simulink model "LRMate200Experimentor_Single"  (R2015b)
settings: Solver=FixedStepDiscrete  StartTime=0.0  StopTime=inf  FixedStep=si.SolverTimeStep  RelTol=1e-3  AbsTol=1e-5
undefined symbols (not defined in the file or in its folder): si
libraries: xpcethercatlib x58, slrtlib x8, xpcnilib x6
settings Model: xpc_rtwmakecfg_data=_xpcethercatlib_  SimulationMode=external  ExtModeTrigDuration=2000  ExtModeTrigDurationFloating=1000  Creator=zwashizu  LastModifiedBy=FANUC
settings SolverCC: EnableConcurrentExecution=on
settings DataIOCC: SaveFormat=Array  Refine=2
settings OptimizationCC: BlockReduction=off  OptimizeBlockIOStorage=off  BufferReuse=off  GlobalBufferReuse=off  ExpressionFolding=off  ExpressionDepthLimit=2147483647  LocalBlockOutputs=off
settings DebuggingCC: AlgebraicLoopMsg=none  ArtificialAlgebraicLoopMsg=none  UnderspecifiedInitializationDetection=Classic  MergeDetectMultiDrivingBlocksExec=none  SolverPrmCheckMsg=warning  MultiTaskDSMMsg=none  FcnCallInpInsideContextMsg=UseLocalSettings  StateNameClashWarn=warning
settings HardwareCC: ProdBitPerPointer=32  ProdLargestAtomicFloat=None  ProdWordSize=32  ProdLongLongMode=on  ProdHWDeviceType=Generic->32-bit x86 compatible
settings RTWCC: SystemTargetFile=slrt.tlc  TemplateMakefile=slrt_default_tmf  Description=Simulink Real-Time  RTWCompilerOptimization=on
settings CodeAppCC: MaxIdLength=120
settings SimulinkRealTimeCC: GeneratePreprocessorConditionals=Disable all
settings ConfigComp: CovModelRefEnable=Off  CovSFcnEnable=off

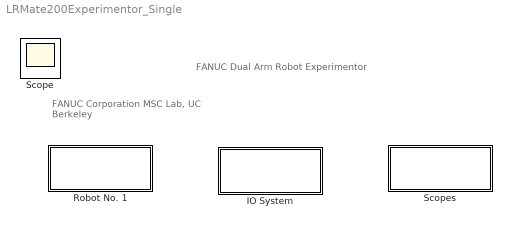
== system LRMate200Experimentor_Single ==
  note: FANUC Dual Arm Robot Experimentor
  note: FANUC Corporation
      | MSC Lab, UC Berkeley
  IO System : Subsystem
  Robot No. 1 : Subsystem
  Scopes : Subsystem
  Scope : Scope

== system LRMate200Experimentor_Single/IO System ==
  note: The Board Bus/Slot Number might be different in different TargetPC
  Button : Subsystem
  DSA System : Subsystem
  "EtherCAT Init " : xpcethercatlib/EtherCAT Init   Priority=0  config_file=F:\TeTang\V4.0\experimentor\ENI_File_20150509_2DSA.xml  device_id=0  pci_bus=3  pci_slot=0  dctuning=0  enaDebug=off  enaDC=on  errLink=off  masterDbg=off  stateChgDbg=on  baseClock=off  masterCfg=off  logFile='c:\dbglog.txt'  sample_time=0.000250
  EtherCAT Init Status : Subsystem
  Force Sensor : Subsystem
  Gripper System : Subsystem
  IO Board Brake Subsystem : Subsystem
  wires:
  "EtherCAT Init "/1 -> EtherCAT Init Status/1(In1)

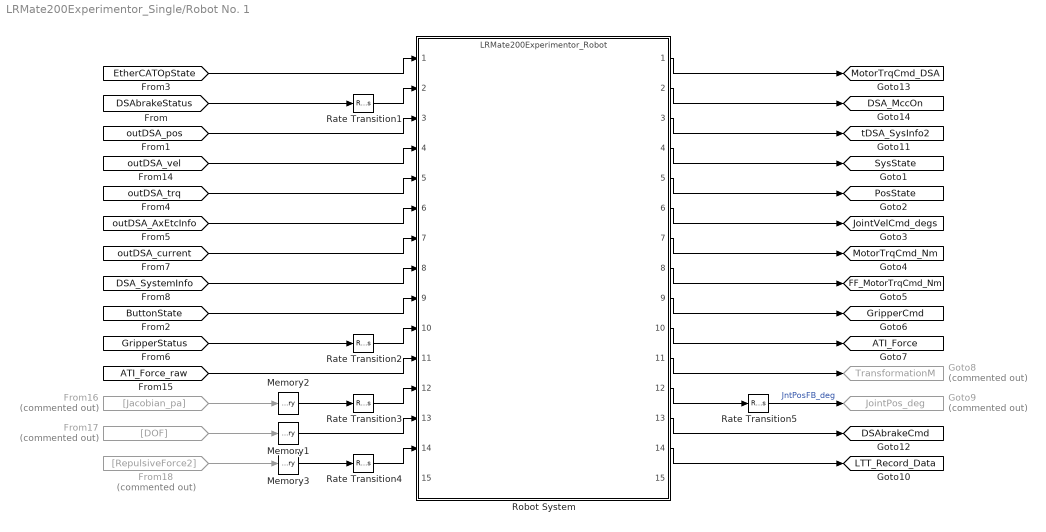
== system LRMate200Experimentor_Single/Robot No. 1 ==
  From16 : From  Commented=on  GotoTag=Jacobian_pa  TagVisibility=global
  From17 : From  Commented=on  GotoTag=DOF  TagVisibility=global
  From18 : From  Commented=on  GotoTag=RepulsiveForce2  TagVisibility=global
  Goto8 : Goto  Commented=on  GotoTag=TransformationM  TagVisibility=global
  Goto9 : Goto  Commented=on  GotoTag=JointPos_deg  TagVisibility=global
  Memory1 : Memory  InheritSampleTime=on
  Memory2 : Memory  InheritSampleTime=on
  Memory3 : Memory  InheritSampleTime=on
  Rate Transition{1..4} (4 alike) : RateTransition
  Rate Transition5 : RateTransition  OutPortSampleTime=si.tsv
  Robot System : ModelReference  ModelNameDialog=LRMate200Experimentor_Robot.slx  ParameterArgumentNames=rsi  ParameterArgumentValues=si.ri{1}  SimulationMode=Normal  ModelReferenceVersion=1.702  CopyOfModelName=LRMate200Experimentor_Robot.slx
  tag scope: ATI_Force=global, DSA_MccOn=global, DSAbrakeCmd=global, FF_MotorTrqCmd_Nm=global, GripperCmd=global, JointVelCmd_degs=global, LTT_Record_Data=global, MotorTrqCmd_DSA=global, MotorTrqCmd_Nm=global, PosState=global, SysState=global, tDSA_SysInfo2=global
  wires:
  [EtherCATOpState] -> Robot System/1
  [DSAbrakeStatus] -> Rate Transition1/1
  [outDSA_pos] -> Robot System/3
  [outDSA_vel] -> Robot System/4
  [outDSA_trq] -> Robot System/5
  [outDSA_AxEtcInfo] -> Robot System/6
  [outDSA_current] -> Robot System/7
  [DSA_SystemInfo] -> Robot System/8
  [ButtonState] -> Robot System/9
  [GripperStatus] -> Rate Transition2/1
  [ATI_Force_raw] -> Robot System/11
  From16/1 -> Memory2/1
  From17/1 -> Memory1/1
  From18/1 -> Memory3/1
  Robot System/13 -> [DSAbrakeCmd]
  Robot System/12 -> Rate Transition5/1
  Robot System/11 -> Goto8/1
  Robot System/10 -> [ATI_Force]
  Robot System/9 -> [GripperCmd]
  Robot System/8 -> [FF_MotorTrqCmd_Nm]
  Robot System/7 -> [MotorTrqCmd_Nm]
  Robot System/6 -> [JointVelCmd_degs]
  Robot System/5 -> [PosState]
  Robot System/4 -> [SysState]
  Robot System/3 -> [tDSA_SysInfo2]
  Robot System/2 -> [DSA_MccOn]
  Robot System/1 -> [MotorTrqCmd_DSA]
  Rate Transition1/1 -> Robot System/2
  Rate Transition2/1 -> Robot System/10
  Rate Transition3/1 -> Robot System/12
  Rate Transition4/1 -> Robot System/14
  Memory3/1 -> Rate Transition4/1
  Memory1/1 -> Robot System/13
  Memory2/1 -> Rate Transition3/1
  Rate Transition5/1 -> Goto9/1  "JntPosFB_deg"
  Robot System/14 -> [LTT_Record_Data]

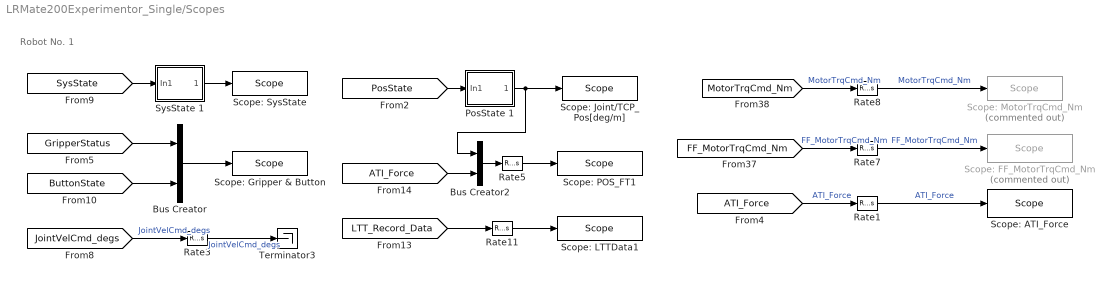
== system LRMate200Experimentor_Single/Scopes ==
  note: Robot No. 1
  Bus Creator : BusCreator  Inputs=2
  Bus Creator2 : BusCreator  Inputs=2
  PosState 1 : Subsystem
  Rate{1,3,5,7..8,11} (6 alike) : RateTransition  OutPortSampleTime=si.tsv
  Scope: ATI_Force : slrtlib/Displays and Logging/Scope   scopeno=7  scopetype=Target  autostart=on  viewmode=Graphical rolling  formatstr='%15.6f'  grid=on  ylimits=[0,0]  nosamples=40000  noprepostsamples=0  interleave=1  triggermode=FreeRun  triggersignal=1  trigsignalfromport=off  triggerlevel=0.0  triggerslope=Either  triggerscope=1  triggersample=0  filename=data.dat  mode=Lazy  writesize=512  autorestart=off  dynamicfilemode=off  maxwritefilesize=512*1024^2
  Scope: FF_MotorTrqCmd_Nm : slrtlib/Displays and Logging/Scope   Commented=on  scopeno=7  scopetype=Target  autostart=on  viewmode=Graphical rolling  formatstr='%15.6f'  grid=on  ylimits=[0,0]  nosamples=40000  noprepostsamples=0  interleave=1  triggermode=FreeRun  triggersignal=1  trigsignalfromport=off  triggerlevel=0.0  triggerslope=Either  triggerscope=1  triggersample=0  filename=data.dat  mode=Lazy  writesize=512  autorestart=off  dynamicfilemode=off  maxwritefilesize=512*1024^2
  Scope: Gripper & Button : slrtlib/Displays and Logging/Scope   scopeno=3  scopetype=Target  autostart=on  viewmode=Numerical  formatstr='%15.6f'  grid=on  ylimits=[0,0]  nosamples=10  noprepostsamples=0  interleave=1  triggermode=FreeRun  triggersignal=1  trigsignalfromport=off  triggerlevel=0.0  triggerslope=Either  triggerscope=1  triggersample=0  filename=data.dat  mode=Lazy  writesize=512  autorestart=off  dynamicfilemode=off  maxwritefilesize=512*1024^2
  Scope: Joint/TCP_Pos[deg/m] : slrtlib/Displays and Logging/Scope   scopeno=2  scopetype=Target  autostart=on  viewmode=Numerical  formatstr='%15.6f'  grid=on  ylimits=[0,0]  nosamples=100  noprepostsamples=0  interleave=1  triggermode=FreeRun  triggersignal=1  trigsignalfromport=off  triggerlevel=0.0  triggerslope=Either  triggerscope=1  triggersample=0  filename=data.dat  mode=Lazy  writesize=512  autorestart=off  dynamicfilemode=off  maxwritefilesize=512*1024^2
  Scope: LTTData1 : slrtlib/Displays and Logging/Scope   scopeno=12  scopetype=File  autostart=on  viewmode=Graphical redraw  formatstr='%15.6f'  grid=on  ylimits=[0,0]  nosamples=si.FileScope_NumberOfSamples  noprepostsamples=0  interleave=1  triggermode=FreeRun  triggersignal=1  trigsignalfromport=off  triggerlevel=0.0  triggerslope=Either  triggerscope=1  triggersample=0  filename=c:LTTData1.dat  mode=Lazy  writesize=512  autorestart=on  dynamicfilemode=off  maxwritefilesize=512*1024^2
  Scope: MotorTrqCmd_Nm : slrtlib/Displays and Logging/Scope   Commented=on  scopeno=3  scopetype=Target  autostart=on  viewmode=Graphical rolling  formatstr='%15.6f'  grid=on  ylimits=[0,0]  nosamples=40000  noprepostsamples=0  interleave=1  triggermode=FreeRun  triggersignal=1  trigsignalfromport=off  triggerlevel=0.0  triggerslope=Either  triggerscope=1  triggersample=0  filename=data.dat  mode=Lazy  writesize=512  autorestart=off  dynamicfilemode=off  maxwritefilesize=512*1024^2
  Scope: POS_FT1 : slrtlib/Displays and Logging/Scope   scopeno=10  scopetype=File  autostart=on  viewmode=Graphical redraw  formatstr='%15.6f'  grid=on  ylimits=[0,0]  nosamples=si.FileScope_NumberOfSamples  noprepostsamples=0  interleave=1  triggermode=FreeRun  triggersignal=1  trigsignalfromport=off  triggerlevel=0.0  triggerslope=Either  triggerscope=1  triggersample=0  filename=c:POS_FT1.dat  mode=Lazy  writesize=512  autorestart=on  dynamicfilemode=off  maxwritefilesize=512*1024^2
  Scope: SysState : slrtlib/Displays and Logging/Scope   scopeno=1  scopetype=Target  autostart=on  viewmode=Numerical  formatstr='%15.6f'  grid=on  ylimits=[0,0]  nosamples=10  noprepostsamples=0  interleave=1  triggermode=FreeRun  triggersignal=1  trigsignalfromport=off  triggerlevel=0.0  triggerslope=Either  triggerscope=1  triggersample=0  filename=data.dat  mode=Lazy  writesize=512  autorestart=off  dynamicfilemode=off  maxwritefilesize=512*1024^2
  SysState 1 : Subsystem
  Terminator3 : Terminator
  wires:
  [PosState] -> PosState 1/1(In1)
  [FF_MotorTrqCmd_Nm] -> Rate7/1  "FF_MotorTrqCmd_Nm"
  Rate7/1 -> Scope: FF_MotorTrqCmd_Nm/1  "FF_MotorTrqCmd_Nm"
  [MotorTrqCmd_Nm] -> Rate8/1  "MotorTrqCmd_Nm"
  Rate8/1 -> Scope: MotorTrqCmd_Nm/1  "MotorTrqCmd_Nm"
  [SysState] -> SysState 1/1(In1)
  SysState 1/1(Out1) -> Scope: SysState/1
  [ATI_Force] -> Rate1/1  "ATI_Force"
  Rate1/1 -> Scope: ATI_Force/1  "ATI_Force"
  [GripperStatus] -> Bus Creator/1
  [ButtonState] -> Bus Creator/2
  Bus Creator/1 -> Scope: Gripper & Button/1
  [JointVelCmd_degs] -> Rate3/1  "JointVelCmd_degs"
  Rate3/1 -> Terminator3/1  "JointVelCmd_degs"
  PosState 1/1(Out1) -> Scope: Joint/TCP_Pos[deg/m]/1, Bus Creator2/1
  [ATI_Force] -> Bus Creator2/2
  Bus Creator2/1 -> Rate5/1
  Rate5/1 -> Scope: POS_FT1/1
  [LTT_Record_Data] -> Rate11/1
  Rate11/1 -> Scope: LTTData1/1

== system LRMate200Experimentor_Single/IO System/Button ==
  Bus Creator : BusCreator  Inputs=2
  PCI-6528 DI Port 1 : xpcnilib/Digital Input/PCI-6528 DI  channel=[5,6]  port=B  filter=[0]  filtertime=0  sample=.001  slot=-1
  tag scope: ButtonState=global
  wires:
  PCI-6528 DI Port 1/1 -> Bus Creator/1  "Green_Button"
  PCI-6528 DI Port 1/2 -> Bus Creator/2  "LTT_Button"
  Bus Creator/1 -> [ButtonState]

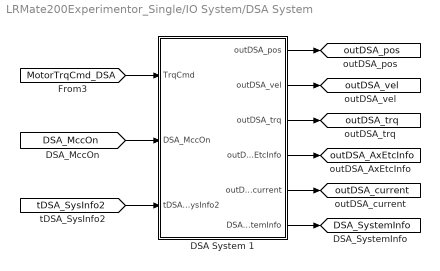
== system LRMate200Experimentor_Single/IO System/DSA System ==
  DSA System 1 : Subsystem
      settings: MinAlgLoopOccurrences=on
  tag scope: DSA_SystemInfo=global, outDSA_AxEtcInfo=global, outDSA_current=global, outDSA_pos=global, outDSA_trq=global, outDSA_vel=global
  wires:
  [MotorTrqCmd_DSA] -> DSA System 1/1(TrqCmd)
  [DSA_MccOn] -> DSA System 1/2(DSA_MccOn)
  [tDSA_SysInfo2] -> DSA System 1/3(tDSA_SysInfo2)
  DSA System 1/1(outDSA_pos) -> [outDSA_pos]
  DSA System 1/2(outDSA_vel) -> [outDSA_vel]
  DSA System 1/3(outDSA_trq) -> [outDSA_trq]
  DSA System 1/4(outDSA_AxEtcInfo) -> [outDSA_AxEtcInfo]
  DSA System 1/5(outDSA_current) -> [outDSA_current]
  DSA System 1/6(DSA_SystemInfo) -> [DSA_SystemInfo]

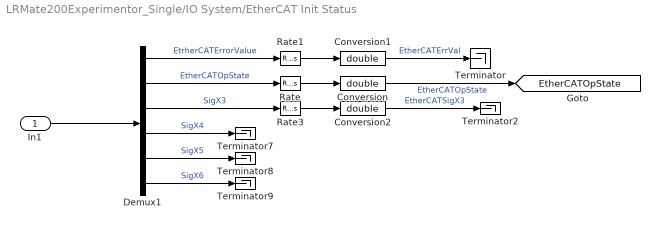
== system LRMate200Experimentor_Single/IO System/EtherCAT Init Status ==
  In1 : Inport
  Conversion : DataTypeConversion  OutDataTypeStr=double
  Conversion1 : DataTypeConversion  OutDataTypeStr=double
  Conversion2 : DataTypeConversion  OutDataTypeStr=double
  Demux1 : Demux  Outputs=6
  Rate : RateTransition  OutPortSampleTime=si.itp
  Rate1 : RateTransition  OutPortSampleTime=si.itp
  Rate3 : RateTransition  OutPortSampleTime=si.itp
  Terminator{,2,7..9} (5 alike) : Terminator
  tag scope: EtherCATOpState=global
  wires:
  Conversion2/1 -> Terminator2/1  "EtherCATSigX3"
  Demux1/4 -> Terminator7/1  "SigX4"
  Demux1/1 -> Rate1/1  "EtrherCATErrorValue"
  Demux1/3 -> Rate3/1  "SigX3"
  Demux1/5 -> Terminator8/1  "SigX5"
  Demux1/2 -> Rate/1  "EtherCATOpState"
  Rate/1 -> Conversion/1
  Rate3/1 -> Conversion2/1
  Conversion/1 -> [EtherCATOpState]  "EtherCATOpState"
  Conversion1/1 -> Terminator/1  "EtherCATErrVal"
  Rate1/1 -> Conversion1/1
  In1/1 -> Demux1/1
  Demux1/6 -> Terminator9/1  "SigX6"

== system LRMate200Experimentor_Single/IO System/Force Sensor ==
  Mux1 : Mux  Inputs=6
  PCI-6259 AD : xpcnilib/A//D/M Series/PCI-6259 AD  channel=[1,2,3,4,5,6]  range=-10*ones(1,6)  coupling=2*ones(1,6)  scantime=5e-6  sampletime=0.001  slot=-1
  tag scope: ATI_Force_raw=global
  wires:
  PCI-6259 AD/3 -> Mux1/3  "Fz(N)"
  Mux1/1 -> [ATI_Force_raw]
  PCI-6259 AD/2 -> Mux1/2  "Fy(N)"
  PCI-6259 AD/6 -> Mux1/6  "Tz(Nm)"
  PCI-6259 AD/4 -> Mux1/4  "Tx(Nm)"
  PCI-6259 AD/5 -> Mux1/5  "Ty(Nm)"
  PCI-6259 AD/1 -> Mux1/1  "Fx(N)"

== system LRMate200Experimentor_Single/IO System/Gripper System ==
  Gripper 1 : Subsystem

== system LRMate200Experimentor_Single/IO System/IO Board Brake Subsystem ==
  PCI-6528 DO : xpcnilib/Digital Output/PCI-6528 DO  channel=[1]  port=A  reset=[1]  initValue=[0]  sample=0.001  slot=-1
  Rate Transition2 : RateTransition  OutPortSampleTime=si.tsv
  tag scope: DSAbrakeStatus=global
  wires:
  [DSAbrakeCmd] -> Rate Transition2/1
  Rate Transition2/1 -> [DSAbrakeStatus], PCI-6528 DO/1  "outDSA_BrakeStatus"

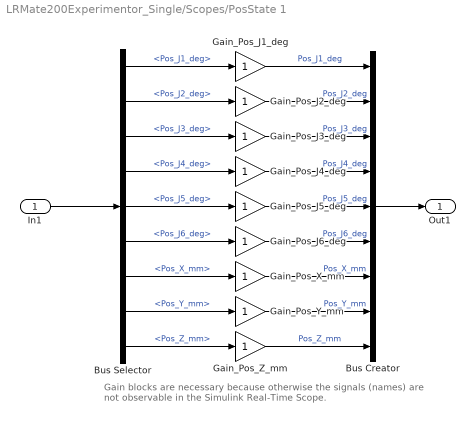
== system LRMate200Experimentor_Single/Scopes/PosState 1 ==
  note: Gain blocks are necessary because otherwise the signals (names) are not observable in the Simulink Real-Time Scope.
  In1 : Inport
  Bus Creator : BusCreator  Inputs=9
  Bus Selector : BusSelector  OutputSignals=Pos_J1_deg,Pos_J2_deg,Pos_J3_deg,Pos_J4_deg,Pos_J5_deg,Pos_J6_deg,Pos_X_mm,Pos_Y_mm,Pos_Z_mm
  Gain_Pos_J1_deg : Gain
  Gain_Pos_J2_deg : Gain
  Gain_Pos_J3_deg : Gain
  Gain_Pos_J4_deg : Gain
  Gain_Pos_J5_deg : Gain
  Gain_Pos_J6_deg : Gain
  Gain_Pos_X_mm : Gain
  Gain_Pos_Y_mm : Gain
  Gain_Pos_Z_mm : Gain
  Out1 : Outport
  wires:
  Bus Creator/1 -> Out1/1
  Bus Selector/1 -> Gain_Pos_J1_deg/1  "<Pos_J1_deg>"
  Bus Selector/2 -> Gain_Pos_J2_deg/1  "<Pos_J2_deg>"
  Bus Selector/3 -> Gain_Pos_J3_deg/1  "<Pos_J3_deg>"
  Bus Selector/4 -> Gain_Pos_J4_deg/1  "<Pos_J4_deg>"
  Bus Selector/5 -> Gain_Pos_J5_deg/1  "<Pos_J5_deg>"
  Bus Selector/6 -> Gain_Pos_J6_deg/1  "<Pos_J6_deg>"
  Bus Selector/7 -> Gain_Pos_X_mm/1  "<Pos_X_mm>"
  Bus Selector/8 -> Gain_Pos_Y_mm/1  "<Pos_Y_mm>"
  Bus Selector/9 -> Gain_Pos_Z_mm/1  "<Pos_Z_mm>"
  In1/1 -> Bus Selector/1
  Gain_Pos_J1_deg/1 -> Bus Creator/1  "Pos_J1_deg"
  Gain_Pos_J2_deg/1 -> Bus Creator/2  "Pos_J2_deg"
  Gain_Pos_J3_deg/1 -> Bus Creator/3  "Pos_J3_deg"
  Gain_Pos_J4_deg/1 -> Bus Creator/4  "Pos_J4_deg"
  Gain_Pos_J5_deg/1 -> Bus Creator/5  "Pos_J5_deg"
  Gain_Pos_J6_deg/1 -> Bus Creator/6  "Pos_J6_deg"
  Gain_Pos_X_mm/1 -> Bus Creator/7  "Pos_X_mm"
  Gain_Pos_Y_mm/1 -> Bus Creator/8  "Pos_Y_mm"
  Gain_Pos_Z_mm/1 -> Bus Creator/9  "Pos_Z_mm"

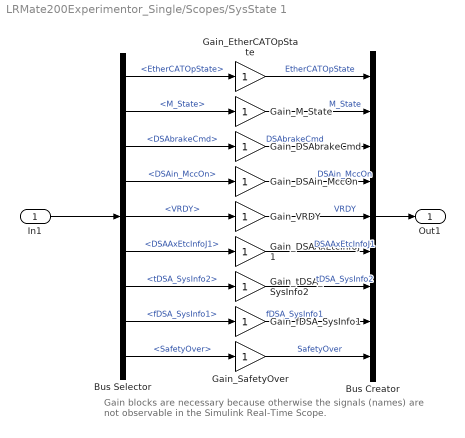
== system LRMate200Experimentor_Single/Scopes/SysState 1 ==
  note: Gain blocks are necessary because otherwise the signals (names) are not observable in the Simulink Real-Time Scope.
  In1 : Inport
  Bus Creator : BusCreator  Inputs=9
  Bus Selector : BusSelector  OutputSignals=EtherCATOpState,M_State,DSAbrakeCmd,DSAin_MccOn,VRDY,DSAAxEtcInfoJ1,tDSA_SysInfo2,fDSA_SysInfo1,SafetyOver
  Gain_DSAAxEtcInfoJ1 : Gain
  Gain_DSAbrakeCmd : Gain
  Gain_DSAin_MccOn : Gain
  Gain_EtherCATOpState : Gain
  Gain_M_State : Gain
  Gain_SafetyOver : Gain
  Gain_VRDY : Gain
  Gain_fDSA_SysInfo1 : Gain
  Gain_tDSA_SysInfo2 : Gain
  Out1 : Outport
  wires:
  Bus Creator/1 -> Out1/1
  Bus Selector/1 -> Gain_EtherCATOpState/1  "<EtherCATOpState>"
  Bus Selector/2 -> Gain_M_State/1  "<M_State>"
  Bus Selector/3 -> Gain_DSAbrakeCmd/1  "<DSAbrakeCmd>"
  Bus Selector/4 -> Gain_DSAin_MccOn/1  "<DSAin_MccOn>"
  Bus Selector/5 -> Gain_VRDY/1  "<VRDY>"
  Bus Selector/6 -> Gain_DSAAxEtcInfoJ1/1  "<DSAAxEtcInfoJ1>"
  Bus Selector/7 -> Gain_tDSA_SysInfo2/1  "<tDSA_SysInfo2>"
  Bus Selector/8 -> Gain_fDSA_SysInfo1/1  "<fDSA_SysInfo1>"
  Bus Selector/9 -> Gain_SafetyOver/1  "<SafetyOver>"
  In1/1 -> Bus Selector/1
  Gain_EtherCATOpState/1 -> Bus Creator/1  "EtherCATOpState"
  Gain_M_State/1 -> Bus Creator/2  "M_State"
  Gain_DSAbrakeCmd/1 -> Bus Creator/3  "DSAbrakeCmd"
  Gain_DSAin_MccOn/1 -> Bus Creator/4  "DSAin_MccOn"
  Gain_VRDY/1 -> Bus Creator/5  "VRDY"
  Gain_DSAAxEtcInfoJ1/1 -> Bus Creator/6  "DSAAxEtcInfoJ1"
  Gain_tDSA_SysInfo2/1 -> Bus Creator/7  "tDSA_SysInfo2"
  Gain_fDSA_SysInfo1/1 -> Bus Creator/8  "fDSA_SysInfo1"
  Gain_SafetyOver/1 -> Bus Creator/9  "SafetyOver"

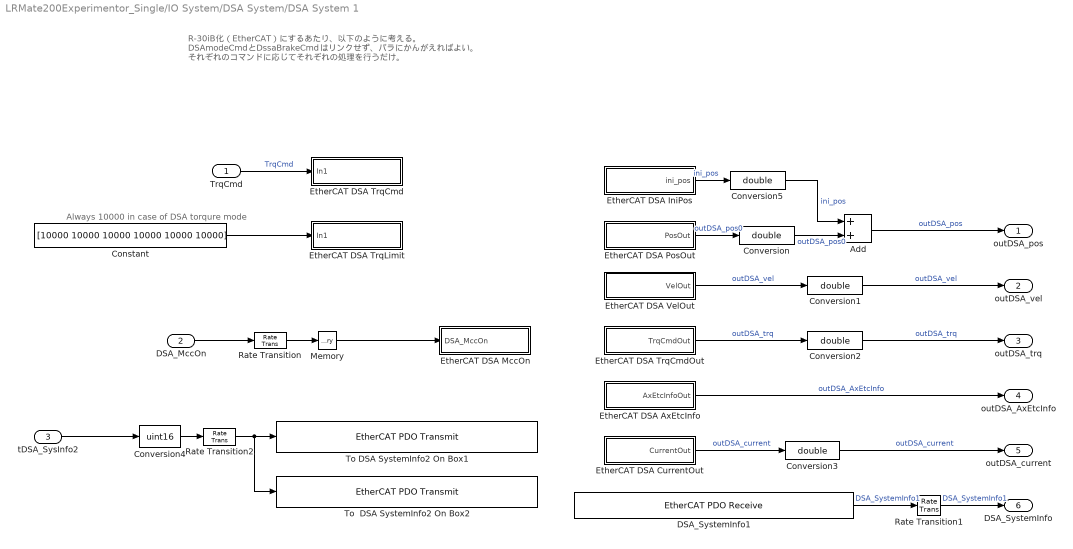
== system LRMate200Experimentor_Single/IO System/DSA System/DSA System 1 ==
  note: Always 10000 in case of DSA torqure mode
  note: R-30iB化（EtherCAT）にするあたり、以下のように考える。
      |
      | DSAmodeCmdとDssaBrakeCmdはリンクせず、パラにかんがえればよい。
      | それぞれのコマンドに応じてそれぞれの処理を行うだけ。
  TrqCmd : Inport
  DSA_MccOn : Inport  Port=2
  tDSA_SysInfo2 : Inport  Port=3
  Add : Sum
  Constant : Constant  Value=[10000 10000 10000 10000 10000 10000]  SampleTime=si.etsv
  Conversion{,1..3,5} (5 alike) : DataTypeConversion  OutDataTypeStr=double
  Conversion4 : DataTypeConversion  OutDataTypeStr=uint16
  DSA_SystemInfo1 : xpcethercatlib/EtherCAT PDO Receive  Priority=2  sig_name=Box 1 (Degital Servo Adapter).NS-IN-SYS-DCIF.NSIS01  sig_offset=1352  sig_type=uint16  type_size=16  sig_dim=1  device_id=0  sample_time=0.000250
  EtherCAT DSA AxEtcInfo : Subsystem
  EtherCAT DSA CurrentOut : Subsystem
  EtherCAT DSA IniPos : Subsystem
  EtherCAT DSA MccOn : Subsystem
  EtherCAT DSA PosOut : Subsystem
  EtherCAT DSA TrqCmd : Subsystem
  EtherCAT DSA TrqCmdOut : Subsystem
  EtherCAT DSA TrqLimit : Subsystem
  EtherCAT DSA VelOut : Subsystem
  Memory : Memory
  Rate Transition : RateTransition
  Rate Transition1 : RateTransition  OutPortSampleTime=si.tsv
  Rate Transition2 : RateTransition
  To  DSA SystemInfo2 On Box2 : xpcethercatlib/EtherCAT PDO Transmit   Priority=3  sig_name=Box 2 (Degital Servo Adapter).NS-OUT-SYS-DCIF.NSOS01  sig_offset=3656  sig_type=uint16  type_size=16  sig_dim=1  device_id=0  sample_time=0.000250
  To DSA SystemInfo2 On Box1 : xpcethercatlib/EtherCAT PDO Transmit   Priority=3  sig_name=Box 1 (Degital Servo Adapter).NS-OUT-SYS-DCIF.NSOS01  sig_offset=1352  sig_type=uint16  type_size=16  sig_dim=1  device_id=0  sample_time=0.000250
  outDSA_pos : Outport
  outDSA_vel : Outport  Port=2
  outDSA_trq : Outport  Port=3
  outDSA_AxEtcInfo : Outport  Port=4
  outDSA_current : Outport  Port=5
  DSA_SystemInfo : Outport  Port=6
  wires:
  EtherCAT DSA VelOut/1(VelOut) -> Conversion1/1  "outDSA_vel"
  EtherCAT DSA PosOut/1(PosOut) -> Conversion/1  "outDSA_pos0"
  EtherCAT DSA TrqCmdOut/1(TrqCmdOut) -> Conversion2/1  "outDSA_trq"
  EtherCAT DSA AxEtcInfo/1(AxEtcInfoOut) -> outDSA_AxEtcInfo/1  "outDSA_AxEtcInfo"
  TrqCmd/1 -> EtherCAT DSA TrqCmd/1(In1)  "TrqCmd"
  Conversion/1 -> Add/2  "outDSA_pos0"
  Conversion1/1 -> outDSA_vel/1  "outDSA_vel"
  Conversion2/1 -> outDSA_trq/1  "outDSA_trq"
  Memory/1 -> EtherCAT DSA MccOn/1(DSA_MccOn)
  Rate Transition/1 -> Memory/1
  EtherCAT DSA CurrentOut/1(CurrentOut) -> Conversion3/1  "outDSA_current"
  Conversion3/1 -> outDSA_current/1  "outDSA_current"
  DSA_MccOn/1 -> Rate Transition/1
  Rate Transition2/1 -> To  DSA SystemInfo2 On Box2/1, To DSA SystemInfo2 On Box1/1
  Conversion4/1 -> Rate Transition2/1
  tDSA_SysInfo2/1 -> Conversion4/1
  EtherCAT DSA IniPos/1(ini_pos) -> Conversion5/1  "ini_pos"
  Conversion5/1 -> Add/1  "ini_pos"
  Add/1 -> outDSA_pos/1  "outDSA_pos"
  DSA_SystemInfo1/1 -> Rate Transition1/1  "DSA_SystemInfo1"
  Constant/1 -> EtherCAT DSA TrqLimit/1(In1)
  Rate Transition1/1 -> DSA_SystemInfo/1  "DSA_SystemInfo1"

== system LRMate200Experimentor_Single/IO System/Gripper System/Gripper 1 ==
  Gripper Subsystem : Subsystem
  tag scope: GripperStatus=global
  wires:
  Gripper Subsystem/1(GripperOutput) -> [GripperStatus]
  [GripperCmd] -> Gripper Subsystem/1(GripperInput)

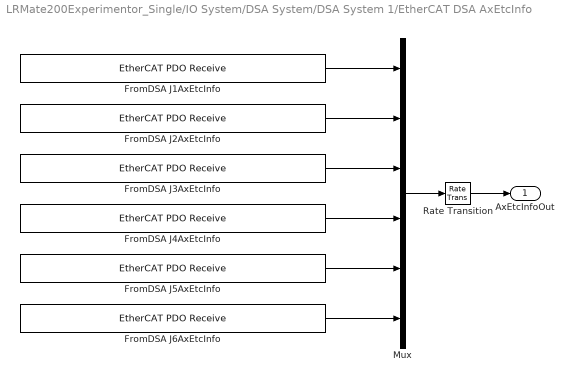
== system LRMate200Experimentor_Single/IO System/DSA System/DSA System 1/EtherCAT DSA AxEtcInfo ==
  FromDSA J1AxEtcInfo : xpcethercatlib/EtherCAT PDO Receive  Priority=2  sig_name=Box 1 (Degital Servo Adapter).NS-IN-AX01.AX01-NSI07  sig_offset=1704  sig_type=uint16  type_size=16  sig_dim=1  device_id=0  sample_time=0.000250
  FromDSA J2AxEtcInfo : xpcethercatlib/EtherCAT PDO Receive  Priority=2  sig_name=Box 1 (Degital Servo Adapter).NS-IN-AX02.AX02-NSI07  sig_offset=1896  sig_type=uint16  type_size=16  sig_dim=1  device_id=0  sample_time=0.000250
  FromDSA J3AxEtcInfo : xpcethercatlib/EtherCAT PDO Receive  Priority=2  sig_name=Box 1 (Degital Servo Adapter).NS-IN-AX03.AX03-NSI07  sig_offset=2088  sig_type=uint16  type_size=16  sig_dim=1  device_id=0  sample_time=0.000250
  FromDSA J4AxEtcInfo : xpcethercatlib/EtherCAT PDO Receive  Priority=2  sig_name=Box 1 (Degital Servo Adapter).NS-IN-AX04.AX04-NSI07  sig_offset=2280  sig_type=uint16  type_size=16  sig_dim=1  device_id=0  sample_time=0.000250
  FromDSA J5AxEtcInfo : xpcethercatlib/EtherCAT PDO Receive  Priority=2  sig_name=Box 2 (Degital Servo Adapter).NS-IN-AX01.AX01-NSI07  sig_offset=4008  sig_type=uint16  type_size=16  sig_dim=1  device_id=0  sample_time=0.000250
  FromDSA J6AxEtcInfo : xpcethercatlib/EtherCAT PDO Receive  Priority=2  sig_name=Box 2 (Degital Servo Adapter).NS-IN-AX02.AX02-NSI07  sig_offset=4200  sig_type=uint16  type_size=16  sig_dim=1  device_id=0  sample_time=0.000250
  Mux : Mux  Inputs=6
  Rate Transition : RateTransition  OutPortSampleTime=si.tsv
  AxEtcInfoOut : Outport
  wires:
  FromDSA J6AxEtcInfo/1 -> Mux/6
  FromDSA J4AxEtcInfo/1 -> Mux/4
  FromDSA J2AxEtcInfo/1 -> Mux/2
  FromDSA J5AxEtcInfo/1 -> Mux/5
  FromDSA J3AxEtcInfo/1 -> Mux/3
  FromDSA J1AxEtcInfo/1 -> Mux/1
  Mux/1 -> Rate Transition/1
  Rate Transition/1 -> AxEtcInfoOut/1

== system LRMate200Experimentor_Single/IO System/DSA System/DSA System 1/EtherCAT DSA CurrentOut ==
  FromDSA J1Current : xpcethercatlib/EtherCAT PDO Receive  Priority=2  sig_name=Box 1 (Degital Servo Adapter).HS-IN-AX01.AX01-HSI03  sig_offset=360  sig_type=int16  type_size=16  sig_dim=1  device_id=0  sample_time=0.000250
  FromDSA J2Current : xpcethercatlib/EtherCAT PDO Receive  Priority=2  sig_name=Box 1 (Degital Servo Adapter).HS-IN-AX02.AX02-HSI03  sig_offset=616  sig_type=int16  type_size=16  sig_dim=1  device_id=0  sample_time=0.000250
  FromDSA J3Current : xpcethercatlib/EtherCAT PDO Receive  Priority=2  sig_name=Box 1 (Degital Servo Adapter).HS-IN-AX03.AX03-HSI03  sig_offset=872  sig_type=int16  type_size=16  sig_dim=1  device_id=0  sample_time=0.000250
  FromDSA J4Current : xpcethercatlib/EtherCAT PDO Receive  Priority=2  sig_name=Box 1 (Degital Servo Adapter).HS-IN-AX04.AX04-HSI03  sig_offset=1128  sig_type=int16  type_size=16  sig_dim=1  device_id=0  sample_time=0.000250
  FromDSA J5Current : xpcethercatlib/EtherCAT PDO Receive  Priority=2  sig_name=Box 2 (Degital Servo Adapter).HS-IN-AX01.AX01-HSI03  sig_offset=2664  sig_type=int16  type_size=16  sig_dim=1  device_id=0  sample_time=0.000250
  FromDSA J6Current : xpcethercatlib/EtherCAT PDO Receive  Priority=2  sig_name=Box 2 (Degital Servo Adapter).HS-IN-AX02.AX02-HSI03  sig_offset=2920  sig_type=int16  type_size=16  sig_dim=1  device_id=0  sample_time=0.000250
  Mux : Mux  Inputs=6
  Rate Transition : RateTransition  OutPortSampleTime=si.tsv
  CurrentOut : Outport
  wires:
  FromDSA J6Current/1 -> Mux/6
  FromDSA J4Current/1 -> Mux/4
  FromDSA J2Current/1 -> Mux/2
  FromDSA J5Current/1 -> Mux/5
  FromDSA J3Current/1 -> Mux/3
  FromDSA J1Current/1 -> Mux/1
  Mux/1 -> Rate Transition/1
  Rate Transition/1 -> CurrentOut/1

== system LRMate200Experimentor_Single/IO System/DSA System/DSA System 1/EtherCAT DSA IniPos ==
  FromDSA J1IniPos : xpcethercatlib/EtherCAT PDO Receive  Priority=2  sig_name=Box 1 (Degital Servo Adapter).NS-IN-AX01.AX01-NSI02  sig_offset=1624  sig_type=int32  type_size=32  sig_dim=1  device_id=0  sample_time=0.000250
  FromDSA J2IniPos : xpcethercatlib/EtherCAT PDO Receive  Priority=2  sig_name=Box 1 (Degital Servo Adapter).NS-IN-AX02.AX02-NSI02  sig_offset=1816  sig_type=int32  type_size=32  sig_dim=1  device_id=0  sample_time=0.000250
  FromDSA J3IniPos : xpcethercatlib/EtherCAT PDO Receive  Priority=2  sig_name=Box 1 (Degital Servo Adapter).NS-IN-AX03.AX03-NSI02  sig_offset=2008  sig_type=int32  type_size=32  sig_dim=1  device_id=0  sample_time=0.000250
  FromDSA J4IniPos : xpcethercatlib/EtherCAT PDO Receive  Priority=2  sig_name=Box 1 (Degital Servo Adapter).NS-IN-AX04.AX04-NSI02  sig_offset=2200  sig_type=int32  type_size=32  sig_dim=1  device_id=0  sample_time=0.000250
  FromDSA J5IniPos : xpcethercatlib/EtherCAT PDO Receive  Priority=2  sig_name=Box 2 (Degital Servo Adapter).NS-IN-AX01.AX01-NSI02  sig_offset=3928  sig_type=int32  type_size=32  sig_dim=1  device_id=0  sample_time=0.000250
  FromDSA J6IniPos : xpcethercatlib/EtherCAT PDO Receive  Priority=2  sig_name=Box 2 (Degital Servo Adapter).NS-IN-AX02.AX02-NSI02  sig_offset=4120  sig_type=int32  type_size=32  sig_dim=1  device_id=0  sample_time=0.000250
  Mux : Mux  Inputs=6
  Rate Transition : RateTransition  OutPortSampleTime=si.tsv
  ini_pos : Outport
  wires:
  FromDSA J6IniPos/1 -> Mux/6
  FromDSA J4IniPos/1 -> Mux/4
  FromDSA J2IniPos/1 -> Mux/2
  FromDSA J5IniPos/1 -> Mux/5
  FromDSA J3IniPos/1 -> Mux/3
  FromDSA J1IniPos/1 -> Mux/1
  Mux/1 -> Rate Transition/1
  Rate Transition/1 -> ini_pos/1

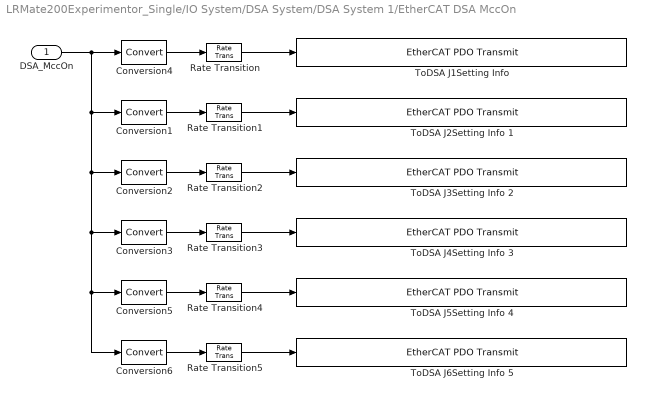
== system LRMate200Experimentor_Single/IO System/DSA System/DSA System 1/EtherCAT DSA MccOn ==
  DSA_MccOn : Inport
  Conversion{1..6} (6 alike) : DataTypeConversion
  Rate Transition{,1..5} (6 alike) : RateTransition
  "ToDSA J1Setting Info " : xpcethercatlib/EtherCAT PDO Transmit   Priority=3  sig_name=Box 1 (Degital Servo Adapter).NS-OUT-AX01.AX01-NSO03  sig_offset=1640  sig_type=uint16  type_size=16  sig_dim=1  device_id=0  sample_time=0.000250
  ToDSA J2Setting Info 1 : xpcethercatlib/EtherCAT PDO Transmit   Priority=3  sig_name=Box 1 (Degital Servo Adapter).NS-OUT-AX02.AX02-NSO03  sig_offset=1896  sig_type=uint16  type_size=16  sig_dim=1  device_id=0  sample_time=0.000250
  ToDSA J3Setting Info 2 : xpcethercatlib/EtherCAT PDO Transmit   Priority=3  sig_name=Box 1 (Degital Servo Adapter).NS-OUT-AX03.AX03-NSO03  sig_offset=2152  sig_type=uint16  type_size=16  sig_dim=1  device_id=0  sample_time=0.000250
  ToDSA J4Setting Info 3 : xpcethercatlib/EtherCAT PDO Transmit   Priority=3  sig_name=Box 1 (Degital Servo Adapter).NS-OUT-AX04.AX04-NSO03  sig_offset=2408  sig_type=uint16  type_size=16  sig_dim=1  device_id=0  sample_time=0.000250
  ToDSA J5Setting Info 4 : xpcethercatlib/EtherCAT PDO Transmit   Priority=3  sig_name=Box 2 (Degital Servo Adapter).NS-OUT-AX01.AX01-NSO03  sig_offset=3944  sig_type=uint16  type_size=16  sig_dim=1  device_id=0  sample_time=0.000250
  ToDSA J6Setting Info 5 : xpcethercatlib/EtherCAT PDO Transmit   Priority=3  sig_name=Box 2 (Degital Servo Adapter).NS-OUT-AX02.AX02-NSO03  sig_offset=4200  sig_type=uint16  type_size=16  sig_dim=1  device_id=0  sample_time=0.000250
  wires:
  Rate Transition/1 -> "ToDSA J1Setting Info "/1
  Conversion4/1 -> Rate Transition/1
  DSA_MccOn/1 -> Conversion6/1, Conversion5/1, Conversion3/1, Conversion2/1, Conversion1/1, Conversion4/1
  Rate Transition1/1 -> ToDSA J2Setting Info 1/1
  Conversion1/1 -> Rate Transition1/1
  Rate Transition2/1 -> ToDSA J3Setting Info 2/1
  Conversion2/1 -> Rate Transition2/1
  Rate Transition3/1 -> ToDSA J4Setting Info 3/1
  Conversion3/1 -> Rate Transition3/1
  Rate Transition4/1 -> ToDSA J5Setting Info 4/1
  Conversion5/1 -> Rate Transition4/1
  Rate Transition5/1 -> ToDSA J6Setting Info 5/1
  Conversion6/1 -> Rate Transition5/1

== system LRMate200Experimentor_Single/IO System/DSA System/DSA System 1/EtherCAT DSA PosOut ==
  FromDSA J1Pos : xpcethercatlib/EtherCAT PDO Receive  Priority=2  sig_name=Box 1 (Degital Servo Adapter).HS-IN-AX01.AX01-HSI12  sig_offset=504  sig_type=int32  type_size=32  sig_dim=1  device_id=0  sample_time=0.000250
  FromDSA J2Pos : xpcethercatlib/EtherCAT PDO Receive  Priority=2  sig_name=Box 1 (Degital Servo Adapter).HS-IN-AX02.AX02-HSI12  sig_offset=760  sig_type=int32  type_size=32  sig_dim=1  device_id=0  sample_time=0.000250
  FromDSA J3Pos : xpcethercatlib/EtherCAT PDO Receive  Priority=2  sig_name=Box 1 (Degital Servo Adapter).HS-IN-AX03.AX03-HSI12  sig_offset=1016  sig_type=int32  type_size=32  sig_dim=1  device_id=0  sample_time=0.000250
  FromDSA J4Pos : xpcethercatlib/EtherCAT PDO Receive  Priority=2  sig_name=Box 1 (Degital Servo Adapter).HS-IN-AX04.AX04-HSI12  sig_offset=1272  sig_type=int32  type_size=32  sig_dim=1  device_id=0  sample_time=0.000250
  FromDSA J5Pos : xpcethercatlib/EtherCAT PDO Receive  Priority=2  sig_name=Box 2 (Degital Servo Adapter).HS-IN-AX01.AX01-HSI12  sig_offset=2808  sig_type=int32  type_size=32  sig_dim=1  device_id=0  sample_time=0.000250
  FromDSA J6Pos : xpcethercatlib/EtherCAT PDO Receive  Priority=2  sig_name=Box 2 (Degital Servo Adapter).HS-IN-AX02.AX02-HSI12  sig_offset=3064  sig_type=int32  type_size=32  sig_dim=1  device_id=0  sample_time=0.000250
  Mux : Mux  Inputs=6
  Rate Transition : RateTransition  OutPortSampleTime=si.tsv
  PosOut : Outport
  wires:
  FromDSA J6Pos/1 -> Mux/6
  FromDSA J4Pos/1 -> Mux/4
  FromDSA J2Pos/1 -> Mux/2
  FromDSA J5Pos/1 -> Mux/5
  FromDSA J3Pos/1 -> Mux/3
  FromDSA J1Pos/1 -> Mux/1
  Mux/1 -> Rate Transition/1
  Rate Transition/1 -> PosOut/1

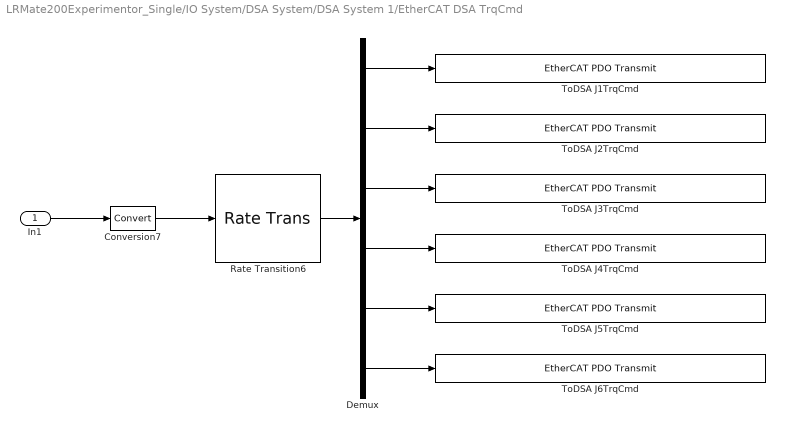
== system LRMate200Experimentor_Single/IO System/DSA System/DSA System 1/EtherCAT DSA TrqCmd ==
  In1 : Inport
  Conversion7 : DataTypeConversion
  Demux : Demux  Outputs=6
  Rate Transition6 : RateTransition
  "ToDSA J1TrqCmd " : xpcethercatlib/EtherCAT PDO Transmit   Priority=3  sig_name=Box 1 (Degital Servo Adapter).HS-OUT-AX01.AX01-HSO04  sig_offset=376  sig_type=int16  type_size=16  sig_dim=1  device_id=0  sample_time=0.000250
  ToDSA J2TrqCmd : xpcethercatlib/EtherCAT PDO Transmit   Priority=3  sig_name=Box 1 (Degital Servo Adapter).HS-OUT-AX02.AX02-HSO04  sig_offset=632  sig_type=int16  type_size=16  sig_dim=1  device_id=0  sample_time=0.000250
  ToDSA J3TrqCmd : xpcethercatlib/EtherCAT PDO Transmit   Priority=3  sig_name=Box 1 (Degital Servo Adapter).HS-OUT-AX03.AX03-HSO04  sig_offset=888  sig_type=int16  type_size=16  sig_dim=1  device_id=0  sample_time=0.000250
  ToDSA J4TrqCmd : xpcethercatlib/EtherCAT PDO Transmit   Priority=3  sig_name=Box 1 (Degital Servo Adapter).HS-OUT-AX04.AX04-HSO04  sig_offset=1144  sig_type=int16  type_size=16  sig_dim=1  device_id=0  sample_time=0.000250
  ToDSA J5TrqCmd : xpcethercatlib/EtherCAT PDO Transmit   Priority=3  sig_name=Box 2 (Degital Servo Adapter).HS-OUT-AX01.AX01-HSO04  sig_offset=2680  sig_type=int16  type_size=16  sig_dim=1  device_id=0  sample_time=0.000250
  ToDSA J6TrqCmd : xpcethercatlib/EtherCAT PDO Transmit   Priority=3  sig_name=Box 2 (Degital Servo Adapter).HS-OUT-AX02.AX02-HSO04  sig_offset=2936  sig_type=int16  type_size=16  sig_dim=1  device_id=0  sample_time=0.000250
  wires:
  In1/1 -> Conversion7/1
  Conversion7/1 -> Rate Transition6/1
  Rate Transition6/1 -> Demux/1
  Demux/1 -> "ToDSA J1TrqCmd "/1
  Demux/2 -> ToDSA J2TrqCmd/1
  Demux/3 -> ToDSA J3TrqCmd/1
  Demux/4 -> ToDSA J4TrqCmd/1
  Demux/5 -> ToDSA J5TrqCmd/1
  Demux/6 -> ToDSA J6TrqCmd/1

== system LRMate200Experimentor_Single/IO System/DSA System/DSA System 1/EtherCAT DSA TrqCmdOut ==
  FromDSA J1TrqCmd : xpcethercatlib/EtherCAT PDO Receive  Priority=2  sig_name=Box 1 (Degital Servo Adapter).HS-IN-AX01.AX01-HSI02  sig_offset=344  sig_type=int16  type_size=16  sig_dim=1  device_id=0  sample_time=0.000250
  FromDSA J2TrqCmd : xpcethercatlib/EtherCAT PDO Receive  Priority=2  sig_name=Box 1 (Degital Servo Adapter).HS-IN-AX02.AX02-HSI02  sig_offset=600  sig_type=int16  type_size=16  sig_dim=1  device_id=0  sample_time=0.000250
  FromDSA J3TrqCmd2 : xpcethercatlib/EtherCAT PDO Receive  Priority=2  sig_name=Box 1 (Degital Servo Adapter).HS-IN-AX03.AX03-HSI02  sig_offset=856  sig_type=int16  type_size=16  sig_dim=1  device_id=0  sample_time=0.000250
  FromDSA J4TrqCmd3 : xpcethercatlib/EtherCAT PDO Receive  Priority=2  sig_name=Box 1 (Degital Servo Adapter).HS-IN-AX04.AX04-HSI02  sig_offset=1112  sig_type=int16  type_size=16  sig_dim=1  device_id=0  sample_time=0.000250
  FromDSA J5TrqCmd4 : xpcethercatlib/EtherCAT PDO Receive  Priority=2  sig_name=Box 2 (Degital Servo Adapter).HS-IN-AX01.AX01-HSI02  sig_offset=2648  sig_type=int16  type_size=16  sig_dim=1  device_id=0  sample_time=0.000250
  FromDSA J6TrqCmd5 : xpcethercatlib/EtherCAT PDO Receive  Priority=2  sig_name=Box 2 (Degital Servo Adapter).HS-IN-AX02.AX02-HSI02  sig_offset=2904  sig_type=int16  type_size=16  sig_dim=1  device_id=0  sample_time=0.000250
  Mux : Mux  Inputs=6
  Rate Transition : RateTransition  OutPortSampleTime=si.tsv
  TrqCmdOut : Outport
  wires:
  FromDSA J6TrqCmd5/1 -> Mux/6
  FromDSA J4TrqCmd3/1 -> Mux/4
  FromDSA J2TrqCmd/1 -> Mux/2
  FromDSA J5TrqCmd4/1 -> Mux/5
  FromDSA J3TrqCmd2/1 -> Mux/3
  FromDSA J1TrqCmd/1 -> Mux/1
  Mux/1 -> Rate Transition/1
  Rate Transition/1 -> TrqCmdOut/1

== system LRMate200Experimentor_Single/IO System/DSA System/DSA System 1/EtherCAT DSA TrqLimit ==
  In1 : Inport
  Conversion7 : DataTypeConversion
  Demux : Demux  Outputs=6
  "ToDSA J1TrqLimit " : xpcethercatlib/EtherCAT PDO Transmit   Priority=3  sig_name=Box 1 (Degital Servo Adapter).HS-OUT-AX01.AX01-HSO05  sig_offset=392  sig_type=int16  type_size=16  sig_dim=1  device_id=0  sample_time=0.000250
  ToDSA J2TrqLimit : xpcethercatlib/EtherCAT PDO Transmit   Priority=3  sig_name=Box 1 (Degital Servo Adapter).HS-OUT-AX02.AX02-HSO05  sig_offset=648  sig_type=int16  type_size=16  sig_dim=1  device_id=0  sample_time=0.000250
  ToDSA J3TrqLimit : xpcethercatlib/EtherCAT PDO Transmit   Priority=3  sig_name=Box 1 (Degital Servo Adapter).HS-OUT-AX03.AX03-HSO05  sig_offset=904  sig_type=int16  type_size=16  sig_dim=1  device_id=0  sample_time=0.000250
  ToDSA J4TrqLimit : xpcethercatlib/EtherCAT PDO Transmit   Priority=3  sig_name=Box 1 (Degital Servo Adapter).HS-OUT-AX04.AX04-HSO05  sig_offset=1160  sig_type=int16  type_size=16  sig_dim=1  device_id=0  sample_time=0.000250
  ToDSA J5TrqLimit : xpcethercatlib/EtherCAT PDO Transmit   Priority=3  sig_name=Box 2 (Degital Servo Adapter).HS-OUT-AX01.AX01-HSO05  sig_offset=2696  sig_type=int16  type_size=16  sig_dim=1  device_id=0  sample_time=0.000250
  ToDSA J6TrqLimit : xpcethercatlib/EtherCAT PDO Transmit   Priority=3  sig_name=Box 2 (Degital Servo Adapter).HS-OUT-AX02.AX02-HSO05  sig_offset=2952  sig_type=int16  type_size=16  sig_dim=1  device_id=0  sample_time=0.000250
  wires:
  In1/1 -> Conversion7/1
  Demux/1 -> "ToDSA J1TrqLimit "/1
  Demux/2 -> ToDSA J2TrqLimit/1
  Demux/3 -> ToDSA J3TrqLimit/1
  Demux/4 -> ToDSA J4TrqLimit/1
  Demux/5 -> ToDSA J5TrqLimit/1
  Demux/6 -> ToDSA J6TrqLimit/1
  Conversion7/1 -> Demux/1

== system LRMate200Experimentor_Single/IO System/DSA System/DSA System 1/EtherCAT DSA VelOut ==
  FromDSA J1Vel : xpcethercatlib/EtherCAT PDO Receive  Priority=2  sig_name=Box 1 (Degital Servo Adapter).HS-IN-AX01.AX01-HSI10  sig_offset=472  sig_type=int32  type_size=32  sig_dim=1  device_id=0  sample_time=0.000250
  FromDSA J2Vel : xpcethercatlib/EtherCAT PDO Receive  Priority=2  sig_name=Box 1 (Degital Servo Adapter).HS-IN-AX02.AX02-HSI10  sig_offset=728  sig_type=int32  type_size=32  sig_dim=1  device_id=0  sample_time=0.000250
  FromDSA J3Vel : xpcethercatlib/EtherCAT PDO Receive  Priority=2  sig_name=Box 1 (Degital Servo Adapter).HS-IN-AX03.AX03-HSI10  sig_offset=984  sig_type=int32  type_size=32  sig_dim=1  device_id=0  sample_time=0.000250
  FromDSA J4Vel : xpcethercatlib/EtherCAT PDO Receive  Priority=2  sig_name=Box 1 (Degital Servo Adapter).HS-IN-AX04.AX04-HSI10  sig_offset=1240  sig_type=int32  type_size=32  sig_dim=1  device_id=0  sample_time=0.000250
  FromDSA J5Vel : xpcethercatlib/EtherCAT PDO Receive  Priority=2  sig_name=Box 2 (Degital Servo Adapter).HS-IN-AX01.AX01-HSI10  sig_offset=2776  sig_type=int32  type_size=32  sig_dim=1  device_id=0  sample_time=0.000250
  FromDSA J6Vel : xpcethercatlib/EtherCAT PDO Receive  Priority=2  sig_name=Box 2 (Degital Servo Adapter).HS-IN-AX02.AX02-HSI10  sig_offset=3032  sig_type=int32  type_size=32  sig_dim=1  device_id=0  sample_time=0.000250
  Mux : Mux  Inputs=6
  Rate Transition : RateTransition  OutPortSampleTime=si.tsv
  VelOut : Outport
  wires:
  FromDSA J6Vel/1 -> Mux/6
  FromDSA J4Vel/1 -> Mux/4
  FromDSA J2Vel/1 -> Mux/2
  FromDSA J5Vel/1 -> Mux/5
  FromDSA J3Vel/1 -> Mux/3
  FromDSA J1Vel/1 -> Mux/1
  Rate Transition/1 -> VelOut/1
  Mux/1 -> Rate Transition/1

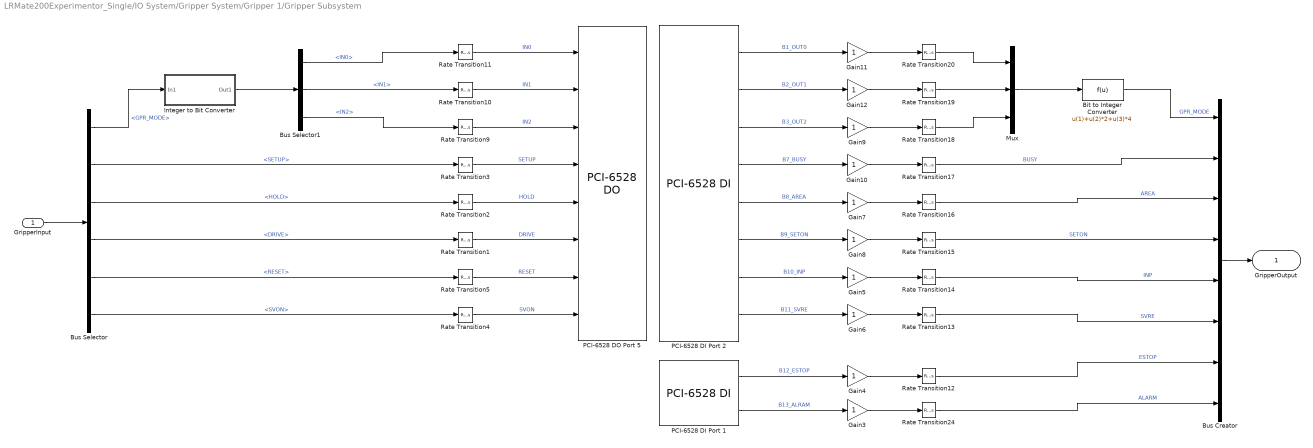
== system LRMate200Experimentor_Single/IO System/Gripper System/Gripper 1/Gripper Subsystem ==
  GripperInput : Inport
  Bit to Integer Converter : Fcn  Expr=u(1)+u(2)*2+u(3)*4
  Bus Creator : BusCreator  Inputs=8
  Bus Selector : BusSelector  OutputSignals=GPR_MODE,SETUP,HOLD,DRIVE,RESET,SVON
  Bus Selector1 : BusSelector  OutputSignals=IN0,IN1,IN2
  Gain{3..12} (10 alike) : Gain
  Integer to Bit Converter : Subsystem  TreatAsAtomicUnit=on
  Mux : Mux  Inputs=3
  PCI-6528 DI Port 1 : xpcnilib/Digital Input/PCI-6528 DI  channel=[8 7]  port=B  filter=[0]  filtertime=0  sample=.001  slot=-1
  PCI-6528 DI Port 2 : xpcnilib/Digital Input/PCI-6528 DI  channel=[8 7 6 5 4 3 2 1]  port=C  filter=[0]  filtertime=0  sample=.001  slot=-1
  PCI-6528 DO Port 5 : xpcnilib/Digital Output/PCI-6528 DO  channel=[8 7 6 5 4 3 2 1]  port=C  reset=[1]  initValue=[0]  sample=0.001  slot=-1
  Rate Transition{1..5,9..20,24} (18 alike) : RateTransition  OutPortSampleTime=si.tsv
  GripperOutput : Outport
  wires:
  Bus Selector/4 -> Rate Transition1/1  "<DRIVE>"
  Rate Transition4/1 -> PCI-6528 DO Port 5/8  "SVON"
  Rate Transition1/1 -> PCI-6528 DO Port 5/6  "DRIVE"
  Rate Transition3/1 -> PCI-6528 DO Port 5/4  "SETUP"
  Bus Selector1/1 -> Rate Transition11/1  "<IN0>"
  Bus Selector1/2 -> Rate Transition10/1  "<IN1>"
  Bus Selector1/3 -> Rate Transition9/1  "<IN2>"
  Bus Selector/2 -> Rate Transition3/1  "<SETUP>"
  Bus Selector/3 -> Rate Transition2/1  "<HOLD>"
  Bus Selector/6 -> Rate Transition4/1  "<SVON>"
  Bus Selector/5 -> Rate Transition5/1  "<RESET>"
  Rate Transition2/1 -> PCI-6528 DO Port 5/5  "HOLD"
  Rate Transition9/1 -> PCI-6528 DO Port 5/3  "IN2"
  Rate Transition10/1 -> PCI-6528 DO Port 5/2  "IN1"
  Rate Transition11/1 -> PCI-6528 DO Port 5/1  "IN0"
  Rate Transition5/1 -> PCI-6528 DO Port 5/7  "RESET"
  GripperInput/1 -> Bus Selector/1
  Gain3/1 -> Rate Transition24/1
  PCI-6528 DI Port 2/6 -> Gain8/1  "B9_SETON"
  Bus Creator/1 -> GripperOutput/1
  Mux/1 -> Bit to Integer Converter/1
  Rate Transition18/1 -> Mux/3
  PCI-6528 DI Port 1/1 -> Gain4/1  "B12_ESTOP"
  PCI-6528 DI Port 2/3 -> Gain9/1  "B3_OUT2"
  PCI-6528 DI Port 2/4 -> Gain10/1  "B7_BUSY"
  Rate Transition20/1 -> Mux/1
  Rate Transition19/1 -> Mux/2
  PCI-6528 DI Port 2/2 -> Gain12/1  "B2_OUT1"
  Gain8/1 -> Rate Transition15/1
  Gain7/1 -> Rate Transition16/1
  PCI-6528 DI Port 2/5 -> Gain7/1  "B8_AREA"
  PCI-6528 DI Port 1/2 -> Gain3/1  "B13_ALRAM"
  Gain11/1 -> Rate Transition20/1
  Gain9/1 -> Rate Transition18/1
  Gain10/1 -> Rate Transition17/1
  Gain12/1 -> Rate Transition19/1
  Gain4/1 -> Rate Transition12/1
  Gain6/1 -> Rate Transition13/1
  PCI-6528 DI Port 2/8 -> Gain6/1  "B11_SVRE"
  PCI-6528 DI Port 2/7 -> Gain5/1  "B10_INP"
  Gain5/1 -> Rate Transition14/1
  PCI-6528 DI Port 2/1 -> Gain11/1  "B1_OUT0"
  Rate Transition16/1 -> Bus Creator/3  "AREA"
  Rate Transition17/1 -> Bus Creator/2  "BUSY"
  Rate Transition15/1 -> Bus Creator/4  "SETON"
  Bit to Integer Converter/1 -> Bus Creator/1  "GPR_MODE"
  Rate Transition13/1 -> Bus Creator/6  "SVRE"
  Rate Transition14/1 -> Bus Creator/5  "INP"
  Rate Transition12/1 -> Bus Creator/7  "ESTOP"
  Rate Transition24/1 -> Bus Creator/8  "ALARM"
  Bus Selector/1 -> Integer to Bit Converter/1(In1)  "<GPR_MODE>"
  Integer to Bit Converter/1(Out1) -> Bus Selector1/1

== system LRMate200Experimentor_Single/IO System/Gripper System/Gripper 1/Gripper Subsystem/Integer to Bit Converter ==
  note: mod(u, 2)
  In1 : Inport
  Bus Creator : BusCreator  Inputs=3
  Fcn : Fcn  Expr=u - 2*floor(u/2)
  Fcn1 : Fcn  Expr=floor(u/2) - 2*floor(floor(u/2)/2)
  Fcn2 : Fcn  Expr=floor(u/4) - 2*floor(floor(u/4)/2)
  Out1 : Outport
  wires:
  In1/1 -> Fcn2/1, Fcn1/1, Fcn/1
  Fcn/1 -> Bus Creator/1  "IN0"
  Fcn1/1 -> Bus Creator/2  "IN1"
  Fcn2/1 -> Bus Creator/3  "IN2"
  Bus Creator/1 -> Out1/1
